simulink model "scout"  (R2018a)
settings: Solver=VariableStepAuto  StartTime=0.0  StopTime=10.0  RelTol=1e-3
undefined symbols (not defined in the file): sigbuilder_block
settings Model: Creator=U500304  LastModifiedBy=U500304

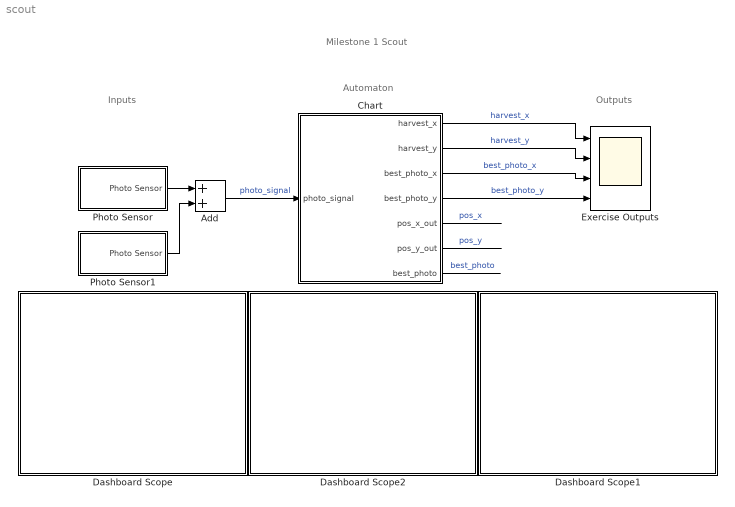
== system scout ==
  note: Outputs
  note: Automaton
  note: Inputs
  note: Milestone 1
      | Scout
  Add : Sum
  Chart : Stateflow chart  TreatAsAtomicUnit=on
  Dashboard Scope : Subsystem  DialogController=hmiCreateDDGDialog  IsWebBlock=on  mask(MWDashboardBlock){webBlockId=c2b4710b-9c10-441f-91da-978dfb24ecfa, webBlockType=sdiscope, ShowInitialText=on, HMISrcModelName=scout}
      mask prompts: webBlockId "WebBlock Id"; webBlockType "WebBlock Type"; HMISrcModelName "Source Model"
      mask help: SimulinkHMI:dialogs:HMIScopeDialogDesc
      mask Help: helpview([docroot '/mapfiles/simulink.map'], 'hmi_scope')
      mask Display:
      | if strcmp(get_param(bdroot(gcb),'BlockDiagramType'), 'library')
      |     image([(matlabroot) '/toolbox/simulink/hmi/icons/DashboardScope.png']);
      | end
  Dashboard Scope1 : Subsystem  DialogController=hmiCreateDDGDialog  IsWebBlock=on  mask(MWDashboardBlock){webBlockId=2d41d672-6b82-41b2-afbb-9518b0dd4a4f, webBlockType=sdiscope, ShowInitialText=on, HMISrcModelName=scout}
      mask prompts: webBlockId "WebBlock Id"; webBlockType "WebBlock Type"; HMISrcModelName "Source Model"
      mask help: SimulinkHMI:dialogs:HMIScopeDialogDesc
      mask Help: helpview([docroot '/mapfiles/simulink.map'], 'hmi_scope')
      mask Display:
      | if strcmp(get_param(bdroot(gcb),'BlockDiagramType'), 'library')
      |     image([(matlabroot) '/toolbox/simulink/hmi/icons/DashboardScope.png']);
      | end
  Dashboard Scope2 : Subsystem  DialogController=hmiCreateDDGDialog  IsWebBlock=on  mask(MWDashboardBlock){webBlockId=ed7f14d0-e4f2-40fb-83fb-68689640cdf1, webBlockType=sdiscope, ShowInitialText=on, HMISrcModelName=scout}
      mask prompts: webBlockId "WebBlock Id"; webBlockType "WebBlock Type"; HMISrcModelName "Source Model"
      mask help: SimulinkHMI:dialogs:HMIScopeDialogDesc
      mask Help: helpview([docroot '/mapfiles/simulink.map'], 'hmi_scope')
      mask Display:
      | if strcmp(get_param(bdroot(gcb),'BlockDiagramType'), 'library')
      |     image([(matlabroot) '/toolbox/simulink/hmi/icons/DashboardScope.png']);
      | end
  Exercise Outputs : Scope  NumInputPorts=4
  Photo Sensor : Subsystem  Tag=STV Subsys  LoadFcn=sigbuilder_block('load');  StartFcn=sigbuilder_block('start');  StopFcn=sigbuilder_block('stop');  ClipboardFcn=sigbuilder_block('clipboard');  mask(Sigbuilder block){tuvar=[0:10]}
      mask help: Simulink:masks:SigbuilderBlock_MD
      mask init:
      | if ~strcmp(get_param(bdroot(gcbh),'SimulationStatus'),'stopped') tuvar = sigbuilder_block('maskInit'); end
      settings: CopyFcn=sigbuilder_block('copy');  DeleteFcn=sigbuilder_block('delete');  ModelCloseFcn=sigbuilder_block('modelClose');  PreSaveFcn=sigbuilder_block('preSave');  PauseFcn=sigbuilder_block('pause');  ContinueFcn=sigbuilder_block('continue');  NameChangeFcn=sigbuilder_block('namechange');  OpenFcn=sigbuilder_block('open',[5.4 30 1141.2 522.6 ]);  CloseFcn=sigbuilder_block('close');
      mask Display: plot(0, 0, 100, 100,[2, 2, 32, 32, 2], [68, 8, 8, 68, 68],[32, 2], [38, 38], [32, 19, 2],[53, 60, 44], [32, 17, 17, 2],[16, 16, 31, 31]);txt = getActiveGroup(gcbh);text(2, 100, txt,'verticalAlignment', 'top');
  Photo Sensor1 : Subsystem  Tag=STV Subsys  LoadFcn=sigbuilder_block('load');  StartFcn=sigbuilder_block('start');  StopFcn=sigbuilder_block('stop');  ClipboardFcn=sigbuilder_block('clipboard');  mask(Sigbuilder block){tuvar=[0:10]}
      mask help: Simulink:masks:SigbuilderBlock_MD
      mask init:
      | if ~strcmp(get_param(bdroot(gcbh),'SimulationStatus'),'stopped') tuvar = sigbuilder_block('maskInit'); end
      settings: CopyFcn=sigbuilder_block('copy');  DeleteFcn=sigbuilder_block('delete');  ModelCloseFcn=sigbuilder_block('modelClose');  PreSaveFcn=sigbuilder_block('preSave');  PauseFcn=sigbuilder_block('pause');  ContinueFcn=sigbuilder_block('continue');  NameChangeFcn=sigbuilder_block('namechange');  OpenFcn=sigbuilder_block('open',[5.4 30 1141.2 522.6 ]);  CloseFcn=sigbuilder_block('close');
      mask Display: plot(0, 0, 100, 100,[2, 2, 32, 32, 2], [68, 8, 8, 68, 68],[32, 2], [38, 38], [32, 19, 2],[53, 60, 44], [32, 17, 17, 2],[16, 16, 31, 31]);txt = getActiveGroup(gcbh);text(2, 100, txt,'verticalAlignment', 'top');
  wires:
  Photo Sensor/1(Photo Sensor) -> Add/1
  Chart/1(harvest_x) -> Exercise Outputs/1  "harvest_x"
  Chart/7(best_photo) -> ?  "best_photo"
  Photo Sensor1/1(Photo Sensor) -> Add/2
  Add/1 -> Chart/1(photo_signal)  "photo_signal"
  Chart/2(harvest_y) -> Exercise Outputs/2  "harvest_y"
  Chart/6(pos_y_out) -> ?  "pos_y"
  Chart/5(pos_x_out) -> ?  "pos_x"
  Chart/3(best_photo_x) -> Exercise Outputs/3  "best_photo_x"
  Chart/4(best_photo_y) -> Exercise Outputs/4  "best_photo_y"

== system scout/Dashboard Scope ==

== system scout/Dashboard Scope1 ==

== system scout/Dashboard Scope2 ==

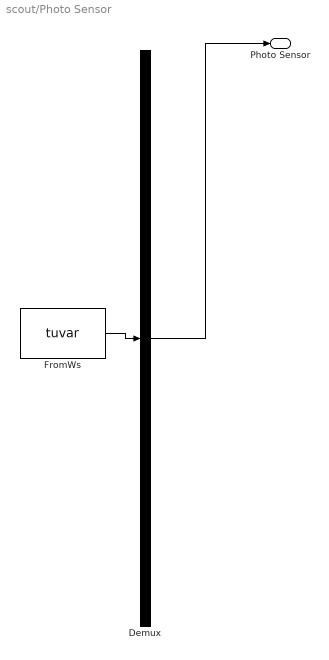
== system scout/Photo Sensor ==
  Demux : Demux  Tag=STV Demux  Outputs=1
  FromWs : FromWorkspace  Tag=STV FromWs  VariableName=tuvar  SampleTime=0
      SigBuilderData=|
      | common.afterFinalStr = 'Extrapolate'
      | common.sampleTime = 0
      | dataSet.timeRange = [0 10]
      | dataSet.name = 'Photo Sensor'
      | sbobj.Groups.Name = 'Photo Sensor'
      | sbobj.Groups.Signals.Name = 'Photo Sensor'
      | sbobj.Groups.Signals.XData = [0 4 4 6 6 10]
      | sbobj.Groups.Signals.YData = [0 0 300 300 0 0]
  Photo Sensor : Outport  Tag=STV Outport
  wires:
  Demux/1 -> Photo Sensor/1
  FromWs/1 -> Demux/1

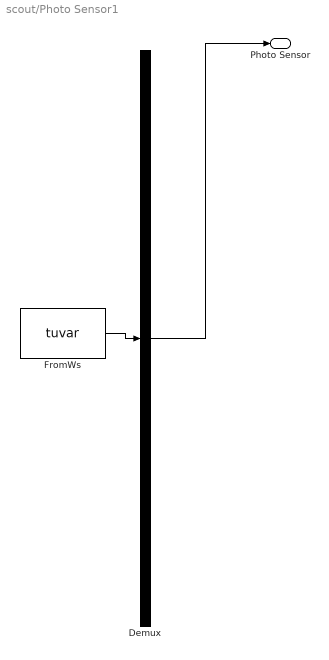
== system scout/Photo Sensor1 ==
  Demux : Demux  Tag=STV Demux  Outputs=1
  FromWs : FromWorkspace  Tag=STV FromWs  VariableName=tuvar  SampleTime=0
      SigBuilderData=|
      | common.afterFinalStr = 'Extrapolate'
      | common.sampleTime = 0
      | dataSet.timeRange = [0 10]
      | dataSet.name = 'Photo Sensor'
      | sbobj.Groups.Name = 'Photo Sensor'
      | sbobj.Groups.Signals.Name = 'Photo Sensor'
      | sbobj.Groups.Signals.XData = [0 1 1 2 2 10]
      | sbobj.Groups.Signals.YData = [0 0 250 250 0 0]
  Photo Sensor : Outport  Tag=STV Outport
  wires:
  FromWs/1 -> Demux/1
  Demux/1 -> Photo Sensor/1

== stateflow chart scout/Chart ==
  settings: updateMethod=CONTINUOUS
  state Drive [parallel]
    settings: executionOrder=1
    state DriveForward
      du:
      pos_x_dot = 1;
      pos_y_dot = 2;
      pos_x_out = pos_x;
      pos_y_out = pos_y;
    (default) -> DriveForward : {
        | pos_x = 0;
        | pos_y = 0'
        | harvest_x = -1;
        | }
  state Sense [parallel]
    settings: executionOrder=2
    state NoLight
    state FoundLight
      en, du:
      harvest_x = pos_x;
      harvest_y = pos_y;
    (default) -> NoLight
    NoLight -> FoundLight : [photo_signal > 200]
    FoundLight -> NoLight [order 2] : [photo_signal <= 200]
    FoundLight -> FoundLight [order 1] : [photo_signal > best_photo]
        | {best_photo = photo_signal;
        | best_photo_x = pos_x;
        | best_photo_y = pos_y;}
  data: harvest_x output; harvest_y output; best_photo_x output; best_photo_y output; pos_x_out output; pos_y_out output; best_photo output =0; pos_x local; pos_y local; photo_signal input
  data pos_x settings: updateMethod=SF_CONTINUOUS_TIME_DATA
  data pos_y settings: updateMethod=SF_CONTINUOUS_TIME_DATA
